simulink model "Nozzle_TestBed1"  (R2019b)
settings: Solver=FixedStepDiscrete  StartTime=0.0  StopTime=1  FixedStep=1  RelTol=1e-3  EnableMultiTasking=on
undefined symbols (not defined in the file): MWS, stripchar_TMATS
libraries: Lib_Turbo_Nozzle_TMATS x1
settings Model: Creator=jwchapm2  LastModifiedBy=bhisma
settings DataIOCC: LimitDataPoints=on  SaveFormat=Array  ReturnWorkspaceOutputs=off
settings OptimizationCC: ExpressionDepthLimit=2147483647  LifeSpan=inf
settings DebuggingCC: UnderspecifiedInitializationDetection=Classic  MergeDetectMultiDrivingBlocksExec=none  SolverPrmCheckMsg=warning  StateNameClashWarn=warning  SFUnexpectedBacktrackingDiag=warning  SFNoUnconditionalDefaultTransitionDiag=warning  SFExecutionAtInitializationDiag=none  ArithmeticOperatorsInVariantConditions=warning
settings HardwareCC: ProdBitPerPointer=32  ProdBitPerSizeT=32  ProdBitPerPtrDiffT=32  ProdLargestAtomicFloat=None  ProdIntDivRoundTo=Undefined  ProdEndianess=Unspecified  ProdWordSize=32  ProdHWDeviceType=32-bit Generic
settings ModelReferenceCC: PropagateSignalLabelsOutOfModel=off
settings SFSimCC: SimUseLocalCustomCode=off  CustomCodeUndefinedFunction=UseInterfaceOnly
settings RTWCC: RTWUseLocalCustomCode=off
settings CodeAppCC: StateflowObjectComments=on
settings GRTTargetCC: TargetLangStandard=C89/C90 (ANSI)  GeneratePreprocessorConditionals=Disable all
settings ConfigComp: CovMetricSettings=dw  CovHtmlReporting=on  CovSaveCumulativeToWorkspaceVar=on  CovSaveSingleToWorkspaceVar=on  CovExternalEMLEnable=off

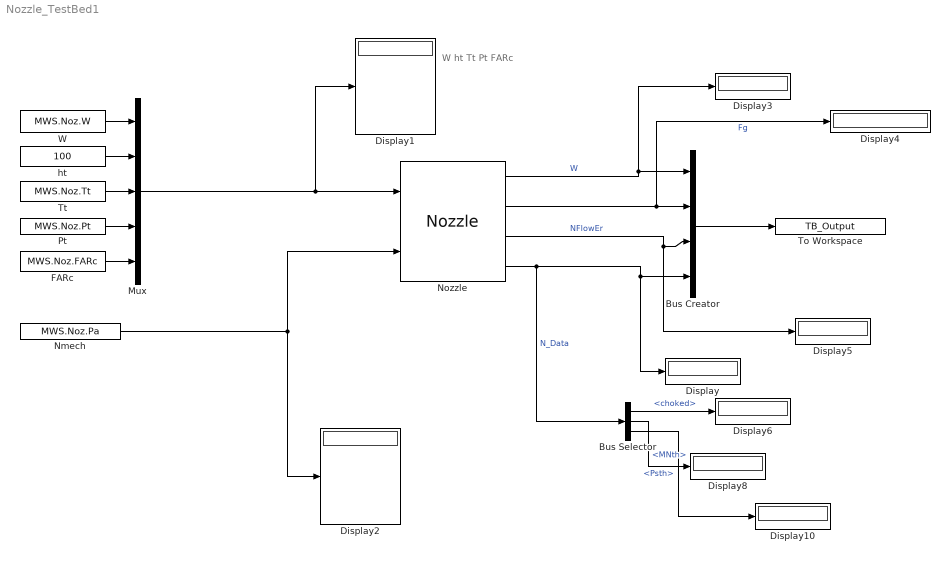
== system Nozzle_TestBed1 ==
  note: W
      | ht
      | Tt
      | Pt
      | FARc
  Bus Selector : BusSelector  OutputSignals=choked,MNth,Psth
  Bus Creator : BusCreator  Inputs=4
  Display{,1..6,8,10} (9 alike) : Display
  FARc : Constant  Value=MWS.Noz.FARc
  Mux : Mux  Inputs=5
  Nmech : Constant  Value=MWS.Noz.Pa
  Nozzle : Lib_Turbo_Nozzle_TMATS/Nozzle  SWType_M=Convergent  N_TArea_M=MWS.Noz.ATh  N_EArea_M=120  N_FL_M=MWS.Noz.LossPerc  X_N_TtVec2_M=MWS.Noz.TtVec  T_N_TGArray_M=MWS.Noz.TGArray  X_N_PEQPaVec_M=MWS.Noz.PeQPaVec  T_N_CdThArray_M=MWS.Noz.CdThArray  T_N_CvArray_M=MWS.Noz.CvArray  CfgEn_M=off  T_N_CfgArray_M=[1 1]  X_N_FARVec_M=MWS.Noz.FARVec  T_N_RtArray_M=MWS.Noz.RArray  Y_N_TtVec_M=MWS.Noz.TtVec  T_N_MAP_gammaArray_M=MWS.Noz.GArray  iDesign_M=2  WDes_M=100  FVar_M=strcat('iDes_',stripchar_TMATS(gcb),'.bin')
  Pt : Constant  Value=MWS.Noz.Pt
  To Workspace : ToWorkspace  VariableName=TB_Output  SampleTime=-1
  Tt : Constant  Value=MWS.Noz.Tt
  W : Constant  Value=MWS.Noz.W
  ht : Constant  Value=100
  wires:
  Nmech/1 -> Display2/1, Nozzle/2
  W/1 -> Mux/1
  FARc/1 -> Mux/5
  Tt/1 -> Mux/3
  Pt/1 -> Mux/4
  Mux/1 -> Display1/1, Nozzle/1
  Nozzle/1 -> Bus Creator/1, Display3/1  "W"
  Nozzle/2 -> Bus Creator/2, Display4/1  "Fg"
  Nozzle/3 -> Bus Creator/3, Display5/1  "NFlowEr"
  Nozzle/4 -> Bus Selector/1, Display/1, Bus Creator/4  "N_Data"
  Bus Creator/1 -> To Workspace/1
  ht/1 -> Mux/2
  Bus Selector/1 -> Display6/1  "<choked>"
  Bus Selector/2 -> Display8/1  "<MNth>"
  Bus Selector/3 -> Display10/1  "<Psth>"
